simulink model "workshop_3link_robot_integration"  (R2022b)
settings: Solver=ode15s  StartTime=0.0  StopTime=30  FixedStep=0.001  RelTol=1e-6  EnableMultiTasking=on
libraries: sm_lib x1
settings Model: Creator=bhorton  LastModifiedBy=kroblet
settings SolverCC: ZeroCrossAlgorithm=Adaptive  AlgebraicLoopSolver=TrustRegion
settings DataIOCC: ReturnWorkspaceOutputs=off
settings OptimizationCC: BlockReduction=off  LifeSpan=inf
settings DebuggingCC: UnconnectedInputMsg=warning  UnconnectedOutputMsg=warning  UnconnectedLineMsg=warning  SFUnexpectedBacktrackingDiag=warning  SFNoUnconditionalDefaultTransitionDiag=warning  SFExecutionAtInitializationDiag=none  SFMachineParentedDataDiag=warning  ArithmeticOperatorsInVariantConditions=warning
settings ModelReferenceCC: EnableRefExpFcnMdlSchedulingChecks=on
settings SFSimCC: SimUseLocalCustomCode=off  CustomCodeUndefinedFunction=UseInterfaceOnly
settings RTWCC: RTWUseLocalCustomCode=off  DLArmComputeVersion=19.05
settings CodeAppCC: StateflowObjectComments=on
settings GRTTargetCC: TargetLangStandard=C89/C90 (ANSI)
settings ConfigComp: CovMetricSettings=dw  CovSaveCumulativeToWorkspaceVar=on  CovSaveSingleToWorkspaceVar=on  CovExternalEMLEnable=off
settings SimscapeCC: SimscapeNormalizeSystem=off  SimscapeLogType=all  SimscapeLogDataHistory=10000
settings ExplorerConfigSet: InternalSimMechanicsExplorerSettings="<ExplorerConfiguration><canonicalview>default</canonicalview><AnimationSetting><BasePlaybackSpeed>1.0</BasePlaybackSpeed><PlaybackSpeedFactor>1.0</PlaybackSpeedFactor></AnimationSetting><TilePanel><TileInfo><Tiles Columns=\"1\" Count=\"1\" Rows=\"1\"><Column Weight=\"1\"/><Row Weight=\"1\"/><Tile Height=\"1\" Width=\"1\" X=\"0\" Y=\"0\"/></Tiles></TileInfo><SceneInfo><SceneViewer><BGColor><R>0.60000002384185791</R><G>0.60000002384185791</G><B>0.60000002384185791</B></BGColor><Camera><DoPerspective>off</DoPerspective><Position><X>0.59337591503002618</X><Y>0.770028921233025243</Y><Z>1.16558506746291179</Z></Position><Center><X>0.554818716269093848</X><Y>0.595850240273192444</Y><Z>-0.00768042407463245119</Z></Center><Up><X>0.010293767731727228</X><Y>0.989057625734068191</Y><Z>-0.147170144129760788</Z></Up><ViewLimDist>1</ViewLimDist><YLim>0.684058578463238476</YLim><XLim>1.00632617542814184</XLim></Camera></SceneViewer></SceneInfo></TilePanel><MechEditorPanel><Cameras/><GfxPanelCameraMap/><VideoCreator><PlaybackSpeedRatio>1.0</PlaybackSpeedRatio><FrameRate>24</FrameRate><VideoFormat>MPEG-4</VideoFormat><FrameSize>[400 400]</FrameSize></VideoCreator></MechEditorPanel></ExplorerConfiguration>"

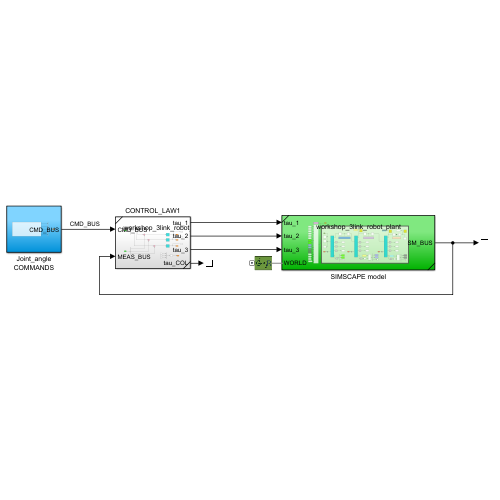
[thumbnail: Simulink's stored preview of the top-level diagram]
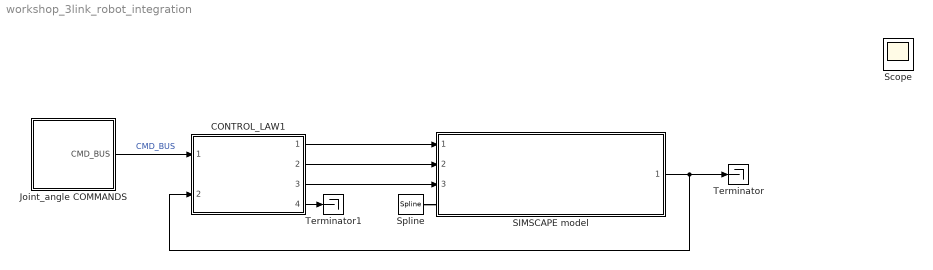
== system workshop_3link_robot_integration ==
  CONTROL_LAW1 : Subsystem  ReferencedSubsystem=workshop_3link_robot_controller
  Joint_angle COMMANDS : Subsystem
  SIMSCAPE model : Subsystem  ReferencedSubsystem=workshop_3link_robot_plant
  Spline : sm_lib/Curves and Surfaces/Spline  GraphicAmbientColor=[0.15 0.15 0.15 1.0]  GraphicDiffuseColor=[0.0 1.0 0.0]  DataPoints=the_EE.XYZ_spline  DataPointsUnits=m  GraphicEmissiveColor=[0.0 0.0 0.0 1.0]  EndConditionType=Natural  MarkerShape=Sphere  MarkerSize=10  GraphicType=FromGeometry  GraphicOpacity=1.0  GraphicShininess=75  GraphicSpecularColor=[0.5 0.5 0.5 1.0]  GraphicVisPropType=SimpleVisualProperties
  Terminator : Terminator
  Terminator1 : Terminator
  Scope : Scope
  wires:
  SIMSCAPE model/1 -> Terminator/1, CONTROL_LAW1/2
  Joint_angle COMMANDS/1(CMD_BUS) -> CONTROL_LAW1/1  "CMD_BUS"
  CONTROL_LAW1/1 -> SIMSCAPE model/1
  CONTROL_LAW1/2 -> SIMSCAPE model/2
  CONTROL_LAW1/3 -> SIMSCAPE model/3
  CONTROL_LAW1/4 -> Terminator1/1
  connections:
  Spline/LConn1 -- SIMSCAPE model/LConn1

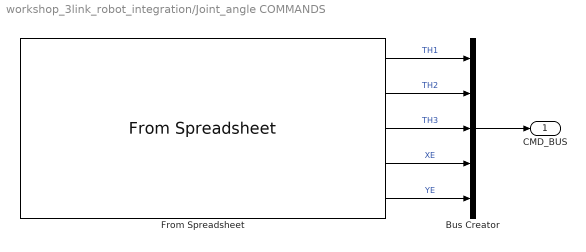
== system workshop_3link_robot_integration/Joint_angle COMMANDS ==
  Bus Creator : BusCreator  Inputs=5
  From Spreadsheet : FromSpreadsheet  FileName=TRAJECTORY_DATA_3LINK.xlsx  SheetName=T_TH_XY  ExtrapolationAfterLastDataPoint=Hold last value
  CMD_BUS : Outport
  wires:
  Bus Creator/1 -> CMD_BUS/1
  From Spreadsheet/1 -> Bus Creator/1  "TH1"
  From Spreadsheet/2 -> Bus Creator/2  "TH2"
  From Spreadsheet/3 -> Bus Creator/3  "TH3"
  From Spreadsheet/4 -> Bus Creator/4  "XE"
  From Spreadsheet/5 -> Bus Creator/5  "YE"
